simulink model "Toy_example_no_names"  (R2024b)
settings: Solver=VariableStepAuto  StartTime=0.0  StopTime=10.0  RelTol=1e-3
settings Model: Creator=Stefania  LastModifiedBy=Stefania

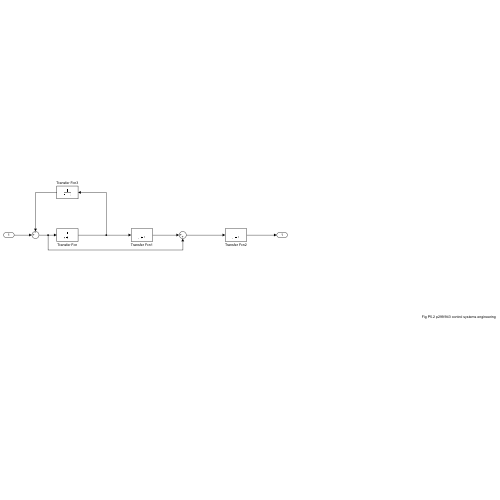
[thumbnail: Simulink's stored preview of the top-level diagram]
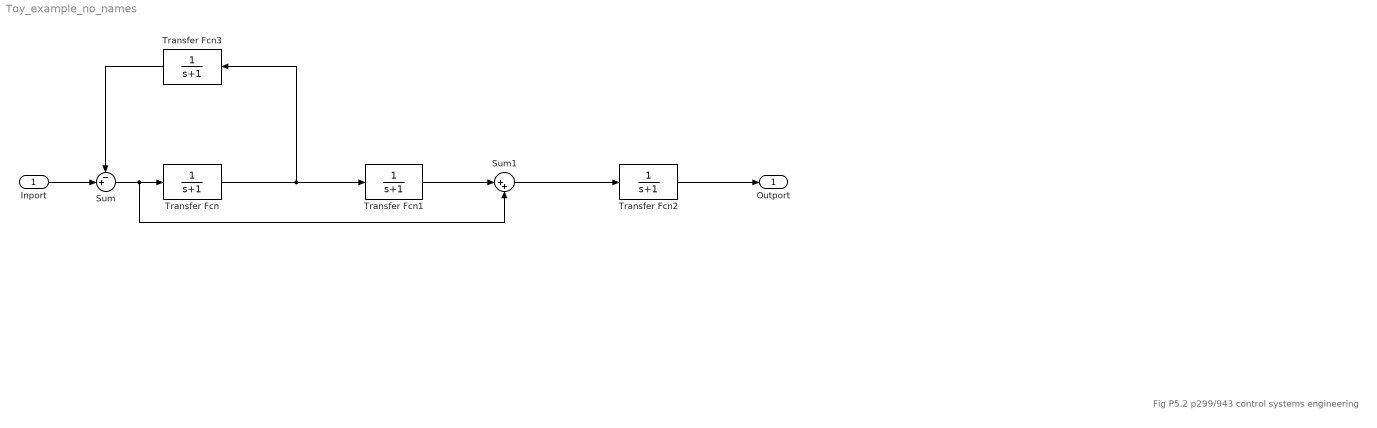
== system Toy_example_no_names ==
  note: Fig P5.2 p299/943 control systems engineering
  Inport : Inport
  Sum : Sum  Inputs=-+|
  Sum1 : Sum  Inputs=|++
  Transfer Fcn{,1..3} (4 alike) : TransferFcn  Denominator=[1 1]
  Outport : Outport
  wires:
  Sum/1 -> Sum1/2, Transfer Fcn/1
  Transfer Fcn/1 -> Transfer Fcn3/1, Transfer Fcn1/1
  Transfer Fcn1/1 -> Sum1/1
  Sum1/1 -> Transfer Fcn2/1
  Transfer Fcn3/1 -> Sum/1
  Inport/1 -> Sum/2
  Transfer Fcn2/1 -> Outport/1
